simulink model "modele_bolide"  (R2023b)
settings: Solver=VariableStepAuto  StartTime=0.0  StopTime=100  RelTol=1e-3
model workspace (MATLAB code in the model file):
  | % Paramètres physiques
  | mb = 1;
  | mw = 1;
  | Ix = 1;
  | Iz = 1;
  | Iwx = 1;
  | Iwy = 1;
  | Iwz = 1;
  | l = 1;
  | d = 1;
  | R = 1;
  | k = 1;
  | rho = 1;
  | 
  | % paramètres à l'équilibre
  | 
  | ybar = 0;
  | ubar = 1;
  | psibar = 0;
  | qbar = 0;
libraries: slpidlib x2

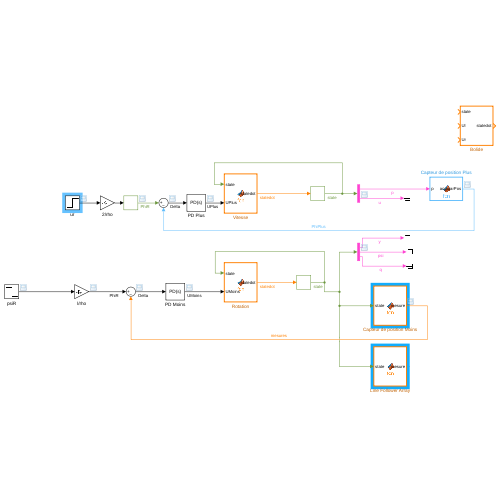
[thumbnail: Simulink's stored preview of the top-level diagram]
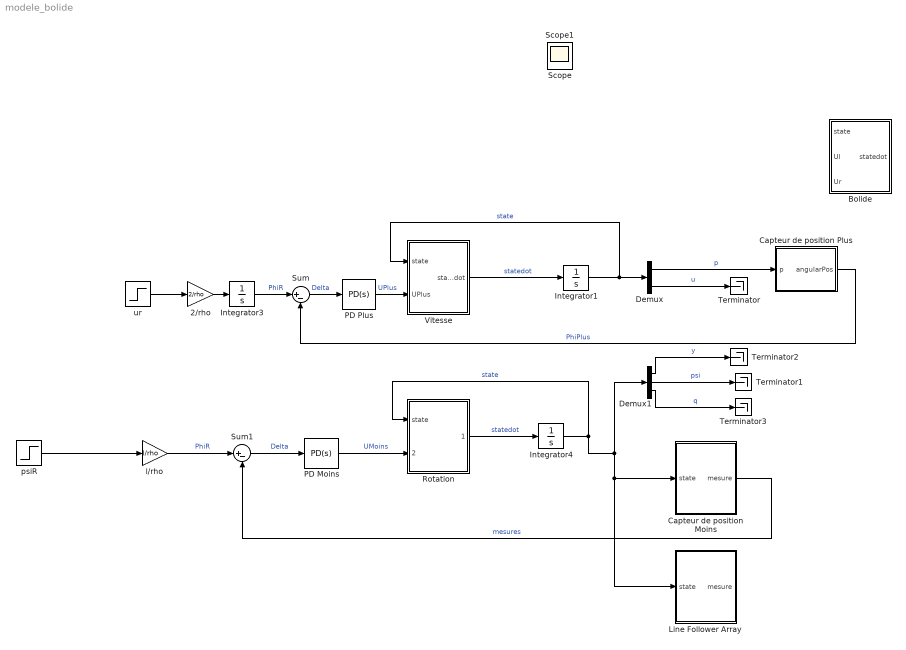
== system modele_bolide ==
  2/rho : Gain  Gain=2/rho
  Bolide : MATLAB Function  TreatAsAtomicUnit=on
  Capteur de position Moins : MATLAB Function  TreatAsAtomicUnit=on
  Capteur de position Plus : MATLAB Function  TreatAsAtomicUnit=on
  Demux : Demux  Outputs=2
  Demux1 : Demux  Outputs=3
  Integrator1 : Integrator
  Integrator3 : Integrator
  Integrator4 : Integrator
  Line Follower Array : MATLAB Function  TreatAsAtomicUnit=on
  PD Moins : slpidlib/PID Controller  Controller=PD  Form=Parallel  TimeDomain=Continuous-time  UseExternalTs=off  SampleTime=-1  IntegratorMethod=Forward Euler  FilterMethod=Forward Euler  ControllerParametersSource=internal  P=11238.494291118  I=1  UseKiTs=off  D=783.815251959048  N=7647.53330101884  UseFilter=on  TunerSelectOption=Transfer Function Based (PID Tuner App)  InitialConditionSource=internal  InitialConditionForIntegrator=0  InitialConditionForFilter=0  DifferentiatorICPrevScaledInput=0  ExternalReset=none  TrackingMode=off  Kt=1  LimitOutput=off  SatLimitsSource=internal  UpperSaturationLimit=inf  LowerSaturationLimit=-inf  LinearizeAsGain=on  AntiWindupMode=none  Kb=1  LimitIntegrator=off  UpperIntegratorSaturationLimit=inf  LowerIntegratorSaturationLimit=-inf  POutMin=[]  POutMax=[]  IOutMin=[]  IOutMax=[]  DOutMin=[]  DOutMax=[]  NOutMin=[]  NOutMax=[]  SumOutMin=[]  SumOutMax=[]  SaturationOutMin=[]  SaturationOutMax=[]  PParamMin=[]  PParamMax=[]  IParamMin=[]  IParamMax=[]  DParamMin=[]  DParamMax=[]  NParamMin=[]  NParamMax=[]  KbParamMin=[]  KbParamMax=[]  KtParamMin=[]  KtParamMax=[]  KbOutMin=[]  KbOutMax=[]  KtOutMin=[]  KtOutMax=[]  IntegratorOutMin=[]  IntegratorOutMax=[]  FilterOutMin=[]  FilterOutMax=[]  SumI1OutMin=[]  SumI1OutMax=[]  SumI2OutMin=[]  SumI2OutMax=[]  SumI3OutMin=[]  SumI3OutMax=[]  SumI4OutMin=[]  SumI4OutMax=[]  SumDOutMin=[]  SumDOutMax=[]  DifferentiatorOutMin=[]  DifferentiatorOutMax=[]  FilterDiffOutCoefMin=[]  FilterDiffOutCoefMax=[]  ReciprocalOutMin=[]  ReciprocalOutMax=[]  SumDenOutMin=[]  SumDenOutMax=[]  SumNumOutMin=[]  SumNumOutMax=[]  DivideOutMin=[]  DivideOutMax=[]  UdiffTsProdOutMin=[]  UdiffTsProdOutMax=[]  NTsProdOutMin=[]  NTsProdOutMax=[]  UintegralTsProdOutMin=[]  UintegralTsProdOutMax=[]  UngainTsProdOutMin=[]  UngainTsProdOutMax=[]  ClampingZeroOutDataTypeStr=Inherit: Inherit via back propagation  ClampingZeroOutMin=[]  ClampingZeroOutMax=[]  FilterDenConstantOutDataTypeStr=Inherit: Inherit via back propagation  FilterDenConstantOutMin=[]  FilterDenConstantOutMax=[]  PCopyOutDataTypeStr=Inherit: Inherit via back propagation  PCopyOutMin=[]  PCopyOutMax=[]  NCopyOutDataTypeStr=Inherit: Inherit via back propagation  NCopyOutMin=[]  NCopyOutMax=[]  IntegratorContinuousStateAttributes=''  IntegratorStateMustResolveToSignalObject=off  IntegratorRTWStateStorageClass=Auto  FilterContinuousStateAttributes=''  FilterStateMustResolveToSignalObject=off  FilterRTWStateStorageClass=Auto  ParallelPVariant=InternalParameters  IdealPVariant=Disabled  IVariant=Disabled  DVariant=InternalParameters  IntegratorVariant=Disabled  SatVariant=Disabled  AWVariant=Disabled  PCopyVariant=Disabled  TRVariant=Disabled  FdbkBlocksVariant=Forward  IdealPFdbkVariant=Disabled  SatFdbkVariant=Disabled  DerivativeFilterVariant=ContFilter  NVariant=InternalParameters  NCopyVariant=Disabled  FilterICVariant=InternalICsFilter  IntegratorICVariant=Disabled  ExternalResetVariant=Disabled  TRSumVariant=Passthrough  SumFdbkVariant=Disabled  SumVariant=Sum_PD  TsampFilterVariant=InternalTs  TsampNgainVariant=Passthrough  TsampIntegralVariant=Disabled_SignalSpec  ExternalSaturationOutDataTypeStr=Inherit: Same as second input
  PD Plus : slpidlib/PID Controller  Controller=PD  Form=Parallel  TimeDomain=Continuous-time  UseExternalTs=off  SampleTime=-1  IntegratorMethod=Forward Euler  FilterMethod=Forward Euler  ControllerParametersSource=internal  P=6.01382806472515  I=1  UseKiTs=off  D=17.8115189243961  N=814.157747769439  UseFilter=on  TunerSelectOption=Transfer Function Based (PID Tuner App)  InitialConditionSource=internal  InitialConditionForIntegrator=0  InitialConditionForFilter=0  DifferentiatorICPrevScaledInput=0  ExternalReset=none  TrackingMode=off  Kt=1  LimitOutput=off  SatLimitsSource=internal  UpperSaturationLimit=inf  LowerSaturationLimit=-inf  LinearizeAsGain=on  AntiWindupMode=none  Kb=1  LimitIntegrator=off  UpperIntegratorSaturationLimit=inf  LowerIntegratorSaturationLimit=-inf  POutMin=[]  POutMax=[]  IOutMin=[]  IOutMax=[]  DOutMin=[]  DOutMax=[]  NOutMin=[]  NOutMax=[]  SumOutMin=[]  SumOutMax=[]  SaturationOutMin=[]  SaturationOutMax=[]  PParamMin=[]  PParamMax=[]  IParamMin=[]  IParamMax=[]  DParamMin=[]  DParamMax=[]  NParamMin=[]  NParamMax=[]  KbParamMin=[]  KbParamMax=[]  KtParamMin=[]  KtParamMax=[]  KbOutMin=[]  KbOutMax=[]  KtOutMin=[]  KtOutMax=[]  IntegratorOutMin=[]  IntegratorOutMax=[]  FilterOutMin=[]  FilterOutMax=[]  SumI1OutMin=[]  SumI1OutMax=[]  SumI2OutMin=[]  SumI2OutMax=[]  SumI3OutMin=[]  SumI3OutMax=[]  SumI4OutMin=[]  SumI4OutMax=[]  SumDOutMin=[]  SumDOutMax=[]  DifferentiatorOutMin=[]  DifferentiatorOutMax=[]  FilterDiffOutCoefMin=[]  FilterDiffOutCoefMax=[]  ReciprocalOutMin=[]  ReciprocalOutMax=[]  SumDenOutMin=[]  SumDenOutMax=[]  SumNumOutMin=[]  SumNumOutMax=[]  DivideOutMin=[]  DivideOutMax=[]  UdiffTsProdOutMin=[]  UdiffTsProdOutMax=[]  NTsProdOutMin=[]  NTsProdOutMax=[]  UintegralTsProdOutMin=[]  UintegralTsProdOutMax=[]  UngainTsProdOutMin=[]  UngainTsProdOutMax=[]  ClampingZeroOutDataTypeStr=Inherit: Inherit via back propagation  ClampingZeroOutMin=[]  ClampingZeroOutMax=[]  FilterDenConstantOutDataTypeStr=Inherit: Inherit via back propagation  FilterDenConstantOutMin=[]  FilterDenConstantOutMax=[]  PCopyOutDataTypeStr=Inherit: Inherit via back propagation  PCopyOutMin=[]  PCopyOutMax=[]  NCopyOutDataTypeStr=Inherit: Inherit via back propagation  NCopyOutMin=[]  NCopyOutMax=[]  IntegratorContinuousStateAttributes=''  IntegratorStateMustResolveToSignalObject=off  IntegratorRTWStateStorageClass=Auto  FilterContinuousStateAttributes=''  FilterStateMustResolveToSignalObject=off  FilterRTWStateStorageClass=Auto  ParallelPVariant=InternalParameters  IdealPVariant=Disabled  IVariant=Disabled  DVariant=InternalParameters  IntegratorVariant=Disabled  SatVariant=Disabled  AWVariant=Disabled  PCopyVariant=Disabled  TRVariant=Disabled  FdbkBlocksVariant=Forward  IdealPFdbkVariant=Disabled  SatFdbkVariant=Disabled  DerivativeFilterVariant=ContFilter  NVariant=InternalParameters  NCopyVariant=Disabled  FilterICVariant=InternalICsFilter  IntegratorICVariant=Disabled  ExternalResetVariant=Disabled  TRSumVariant=Passthrough  SumFdbkVariant=Disabled  SumVariant=Sum_PD  TsampFilterVariant=InternalTs  TsampNgainVariant=Passthrough  TsampIntegralVariant=Disabled_SignalSpec  ExternalSaturationOutDataTypeStr=Inherit: Same as second input
  Rotation : MATLAB Function  TreatAsAtomicUnit=on
  Sum : Sum  Inputs=|+-
  Sum1 : Sum  Inputs=|+-
  Terminator{,1..3} (4 alike) : Terminator
  Vitesse : MATLAB Function  TreatAsAtomicUnit=on
  l/rho : Gain  Gain=l/rho
  psiR : Step  Time=5  Before=20  After=0  SampleTime=0
  ur : Step  Time=5  SampleTime=0
  Scope : Scope
  Scope1 : Scope
  wires:
  Demux/1 -> Capteur de position Plus/1(p)  "p"
  Demux/2 -> Terminator/1  "u"
  Vitesse/1(statedot) -> Integrator1/1  "statedot"
  Integrator1/1 -> Vitesse/1(state), Demux/1  "state"
  PD Plus/1 -> Vitesse/2(UPlus)  "UPlus"
  2/rho/1 -> Integrator3/1
  ur/1 -> 2/rho/1
  Sum/1 -> PD Plus/1  "Delta"
  Capteur de position Plus/1(angularPos) -> Sum/2  "PhiPlus"
  Integrator3/1 -> Sum/1  "PhiR"
  Rotation/1(statedot) -> Integrator4/1  "statedot"
  Integrator4/1 -> Demux1/1, Line Follower Array/1(state), Capteur de position Moins/1(state), Rotation/1(state)  "state"
  Demux1/1 -> Terminator2/1  "y"
  Demux1/2 -> Terminator1/1  "psi"
  Demux1/3 -> Terminator3/1  "q"
  Capteur de position Moins/1(mesure) -> Sum1/2  "mesures"
  PD Moins/1 -> Rotation/2(UMoins)  "UMoins"
  Sum1/1 -> PD Moins/1  "Delta"
  l/rho/1 -> Sum1/1  "PhiR"
  psiR/1 -> l/rho/1

== matlab function modele_bolide/Line Follower Array ==
  data: state input size=[3 1]; mesure output; mb parameter; mw parameter; Ix parameter; Iz parameter; Iwx parameter; Iwy parameter; Iwz parameter; l parameter; d parameter; R parameter; k parameter; rho parameter
function mesure = fcn(state, mb, mw, Ix, Iz, Iwx, Iwy, Iwz, l, d, R, k, rho)

y = state(1);
psi = state(2);
q = state(3);

% Ecritures simplifiées
M = mb + 2*mw;
Ipsi = Ix + Iwx + Iz + Iwz + mw*((l*l)/2) + Iwy*(l*l)/(2*rho*rho);
alpha = M + 2*Iwy/(rho*rho);
beta = Ipsi + mb*d*d;
mu1 = (l*k)/(2*beta*rho*R);
mu2 = (mb*d)/beta;
mu3 = k/(alpha*rho*R);
mu4 = (mb*d)/alpha;


% Equations de fonctionnement

ym = y/cos(psi);

mesure = -ym;

== matlab function modele_bolide/Capteur de position Plus ==
  data: p input; angularPos output; rho parameter
function angularPos = fcn(p,rho)

phiPlus = (2*p)/rho;

angularPos = phiPlus;

== matlab function modele_bolide/Bolide ==
  data: state input size=[6 1]; statedot output; Ul input; Ur input; mb parameter; mw parameter; Ix parameter; Iz parameter; Iwx parameter; Iwy parameter; Iwz parameter; l parameter; d parameter; R parameter; k parameter; rho parameter
function statedot = fcn(state, Ul, Ur, mb, mw, Ix, Iz, Iwx, Iwy, Iwz, l, d, R, k, rho)

% Variables d'état
x = state(1);
y = state(2);
psi = state(3);
q = state(4);
u = state(5);
p = state(6);

% Ecritures simplifiées
M = mb + 2*mw;
Ipsi = Ix + Iwx + Iz + Iwz + mw*((l*l)/2) + Iwy*(l*l)/(2*rho*rho);
alpha = M + 2*Iwy/(rho*rho);
beta = Ipsi + mb*d*d;
mu1 = (l*k)/(2*beta*rho*R);
mu2 = (mb*d)/beta;
mu3 = k/(alpha*rho*R);
mu4 = (mb*d)/alpha;


% Equations de fonctionnement
xdot = u*cos(psi);
ydot = u*sin(psi);
psidot = q;
qdot = mu1*(Ur-Ul-(k*l*q)/rho) + mu2*u*q;
udot = mu3*(Ur+Ul-(2*k*u)/rho) - mu4*q*q;
pdot = u;

statedot = [xdot; ydot; psidot; qdot; udot; pdot];

== matlab function modele_bolide/Rotation ==
  data: state input size=[3 1]; statedot output; UMoins input; mb parameter; mw parameter; Ix parameter; Iz parameter; Iwx parameter; Iwy parameter; Iwz parameter; l parameter; d parameter; R parameter; k parameter; rho parameter; ubar parameter
function statedot = fcn(state, UMoins, mb, mw, Ix, Iz, Iwx, Iwy, Iwz, l, d, R, k, rho, ubar)

% Variables d'état
y = state(1);
psi = state(2);
q = state(3);

% Ecritures simplifiées
M = mb + 2*mw;
Ipsi = Ix + Iwx + Iz + Iwz + mw*((l*l)/2) + Iwy*(l*l)/(2*rho*rho);
alpha = M + 2*Iwy/(rho*rho);
beta = Ipsi + mb*d*d;
mu1 = (l*k)/(2*beta*rho*R);
mu2 = (mb*d)/beta;
mu3 = k/(alpha*rho*R);
mu4 = (mb*d)/alpha;


% Equations de fonctionnement

ydot = ubar*psi;
psidot = q;
qdot = mu1*(UMoins - (k*l*q)/rho) + mu2*ubar*q;

statedot = [ydot; psidot; qdot];

== matlab function modele_bolide/Vitesse ==
  data: state input size=[2 1]; statedot output; UPlus input; mb parameter; mw parameter; Ix parameter; Iz parameter; Iwx parameter; Iwy parameter; Iwz parameter; l parameter; d parameter; R parameter; k parameter; rho parameter
function statedot = fcn(state, UPlus, mb, mw, Ix, Iz, Iwx, Iwy, Iwz, l, d, R, k, rho)

% Variables d'état
p = state(1);
u = state(2);

% Ecritures simplifiées
M = mb + 2*mw;
Ipsi = Ix + Iwx + Iz + Iwz + mw*((l*l)/2) + Iwy*(l*l)/(2*rho*rho);
alpha = M + 2*Iwy/(rho*rho);
beta = Ipsi + mb*d*d;
mu1 = (l*k)/(2*beta*rho*R);
mu2 = (mb*d)/beta;
mu3 = k/(alpha*rho*R);
mu4 = (mb*d)/alpha;


% Equations de fonctionnement

udot = mu3*(UPlus-(2*k*u)/rho);
pdot = u;

statedot = [pdot; udot];

== matlab function modele_bolide/Capteur de position Moins ==
  data: state input size=[3 1]; mesure output; mb parameter; mw parameter; Ix parameter; Iz parameter; Iwx parameter; Iwy parameter; Iwz parameter; l parameter; d parameter; R parameter; k parameter; rho parameter
function mesure = fcn(state, mb, mw, Ix, Iz, Iwx, Iwy, Iwz, l, d, R, k, rho)

y = state(1);
psi = state(2);
q = state(3);

% Ecritures simplifiées
M = mb + 2*mw;
Ipsi = Ix + Iwx + Iz + Iwz + mw*((l*l)/2) + Iwy*(l*l)/(2*rho*rho);
alpha = M + 2*Iwy/(rho*rho);
beta = Ipsi + mb*d*d;
mu1 = (l*k)/(2*beta*rho*R);
mu2 = (mb*d)/beta;
mu3 = k/(alpha*rho*R);
mu4 = (mb*d)/alpha;


% Equations de fonctionnement

PhiMoins = (l*psi)/rho;

mesure = PhiMoins;
